simulink library "INT_CoVM_TrqAcsCoord"  (R2016b)
settings: Solver=VariableStepAuto  StartTime=0.0  StopTime=10.0  RelTol=1e-3
settings Model: Creator=Administrator  LastModifiedBy=Administrator

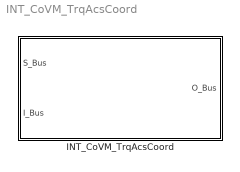
== system INT_CoVM_TrqAcsCoord ==
  INT_CoVM_TrqAcsCoord : Subsystem

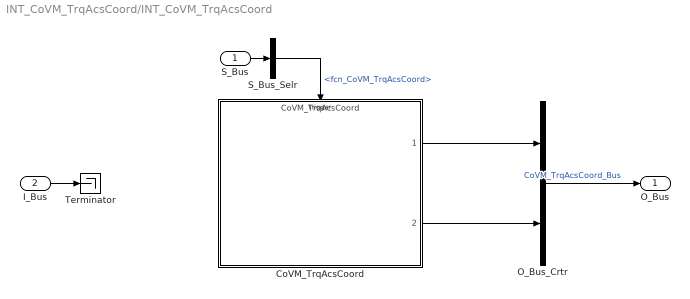
== system INT_CoVM_TrqAcsCoord/INT_CoVM_TrqAcsCoord ==
  S_Bus : Inport
  I_Bus : Inport  Port=2
  CoVM_TrqAcsCoord : ModelReference  ModelNameDialog=CoVM_TrqAcsCoord  SimulationMode=Normal  ModelReferenceVersion=1.3  TriggerPortName=function  TriggerPortTriggerType=function-call  TriggerPortStatesWhenEnabling=held
  O_Bus_Crtr : BusCreator  Inputs=2
  S_Bus_Selr : BusSelector  OutputSignals=fcn_CoVM_TrqAcsCoord
  Terminator : Terminator
  O_Bus : Outport
  wires:
  S_Bus_Selr/1 -> CoVM_TrqAcsCoord/Trigger  "<fcn_CoVM_TrqAcsCoord>"
  S_Bus/1 -> S_Bus_Selr/1
  I_Bus/1 -> Terminator/1
  O_Bus_Crtr/1 -> O_Bus/1  "CoVM_TrqAcsCoord_Bus"
  CoVM_TrqAcsCoord/1 -> O_Bus_Crtr/1
  CoVM_TrqAcsCoord/2 -> O_Bus_Crtr/2
